simulink model "qvmbocsh41_od_2"  (Simulink 5.0)
settings: Solver=ode45  StartTime=0.0  StopTime=5.0  MaxStep=0.001  RelTol=1e-4
undefined symbols (not defined in the file or in its folder): Z10
libraries: simulink_extras x7, dtlib x1
settings Model: LastModifiedBy=krangelo

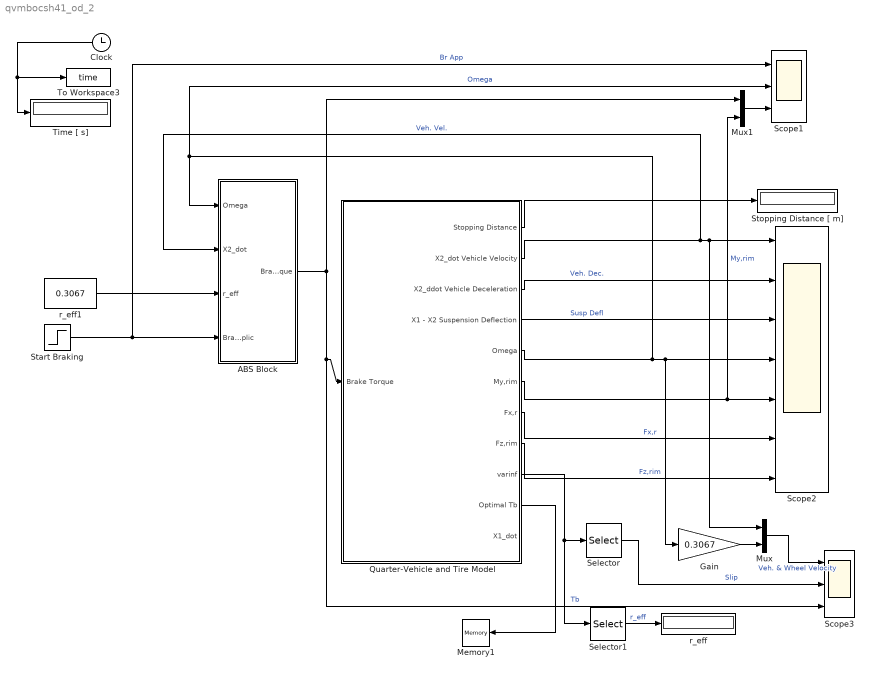
== system qvmbocsh41_od_2 ==
  ABS Block : Subsystem  mask{R1=19000, R2=19000, Bmax=2500, TO=0.0065, TC=0.050, Slip=20, Slipmin=17, neg_a=60, pos_a=3, A=10, om_dot_om=3.5}
      mask prompts: R1 "R1 - Rate of incerase of the  Breake Torque. [Nm/s]"; R2 "R2 - Rate of decerase of the  Breake Torque. [Nm/s]"; Bmax "Bmax - Max. Value of the Brake Torque. [Nm]"; TO "TO - Inlet Valve open time [s]"; TC "TC - Inlet Valve close time [s]"; Slip "Desired slip [%]"; Slipmin "Slipmin - Minimum slip level"; neg_a "-a - Threshold value of the wheel peripheral deceleration [m/s^2]"; pos_a "+a - Threshold value of the wheel peripheral acceleration [m/s^2]"; A "A - Threshold value of the wheel peripheral acceleration [m/s^2]"; om_dot_om "Omdot/Omega -Threshold value of the ratio Om_dot / Om [Hz]"
  Clock : Clock
      settings: Decimation=10
  Gain : Gain  Gain=0.3067  SaturateOnIntegerOverflow=on
  Memory1 : Memory  Orientation=left  X0=0.65
  Mux : Mux  Inputs=2
  Mux1 : Mux  Inputs=2
  Quarter-Vehicle and Tire Model : Subsystem  mask{m2=300, m1=35, kz=20000, Cz=2000, kx=80000, Cx=1100, Vstop=1, Ip=1.04, ro=0.3135, r_eff=0.3067, Vin=80/3.6}
      mask prompts: m2 "m2 - Quarter of the vehicle mass [kg]"; m1 "m1 - Axle mass [kg]"; kz "kz - Suspension stiffness [N/m]"; Cz "cz - Suspension damping [N.s/m]"; kx "kx - Longitudinal suspension stiffness [N/m]"; Cx "cx - Longitudinal suspension damping [N.s/m]"; Vstop "Vstop - Velocity at which the vehicle is considered stoped [m/s]"; Ip "Ip - Wheel polar moment of inertia [kg.m^2]"; ro "ro - Unloaded tire radius [m]"; r_eff "r_eff - Effecive rolling radius [m]"; Vin "Vin - Initial vehicle velocity [m/s]"
      mask help: Vstop - The velocity value, at which the vehicle is considered stoped.
      mask init:
      | disp('initial conditions...')
      | Z10=ro - 9.81*(m1+m2)/195000
      | Z20=Z10 - 9.81*m2/kz
      | X20=0
      | X10=X20+0.01
      | Vin
      | r_eff
      | Om_in=Vin/r_eff
  Scope1 : Scope  NumInputPorts=3
      settings: YMin=0~0~0  YMax=1~95~20000
  Scope2 : Scope  NumInputPorts=7
      settings: TimeRange=5  YMin=21.1325~-1.75e-005~-7e-008~68.8999~0.00025~-0.006~3286.34  YMax=23.3569~0~-6.61744e-024~76.1525~0.00175~0~3286.35  SaveName=ScopeData4
  Scope3 : Scope  NumInputPorts=3
      settings: TimeRange=3  YMin=13.5~-0.225~0  YMax=22.5~0.025~1300  SaveName=ScopeData3
  Selector : Selector  Elements=2  InputPortWidth=40
  Selector1 : Selector  Elements=12  InputPortWidth=40
  Start Braking : Step  Time=2.5  SampleTime=0
  Stopping Distance [ m] : Display
  Time [ s] : Display
  To Workspace3 : ToWorkspace  VariableName=time  SaveFormat=Array
      settings: MaxDataPoints=10000
  r_eff : Display
  r_eff1 : Constant  Value=0.3067
  wires:
  Clock/1 -> Time [ s]/1, To Workspace3/1
  Start Braking/1 -> Scope1/1, ABS Block/4(Brake Applic)  "Br App"
  Quarter-Vehicle and Tire Model/1(Stopping Distance) -> Stopping Distance [ m]/1
  Quarter-Vehicle and Tire Model/5(Omega) -> Scope1/2, ABS Block/1(Omega), Scope2/4, Gain/1  "Omega"
  Quarter-Vehicle and Tire Model/4("X1 - X2 Suspension Deflection ") -> Scope2/3  "Susp Defl"
  Quarter-Vehicle and Tire Model/3(X2_ddot Vehicle Deceleration) -> Scope2/2  "Veh. Dec."
  Quarter-Vehicle and Tire Model/8(Fz,rim) -> Scope2/7  "Fz,rim"
  Quarter-Vehicle and Tire Model/6(My,rim) -> Scope2/5, Mux1/2  "My,rim"
  Quarter-Vehicle and Tire Model/2(X2_dot Vehicle Velocity) -> Scope2/1, Mux/1, ABS Block/2(X2_dot)  "Veh. Vel."
  Quarter-Vehicle and Tire Model/7(Fx,r) -> Scope2/6  "Fx,r"
  ABS Block/1(Brake Torque) -> Scope3/3, Quarter-Vehicle and Tire Model/1(" Brake Torque"), Mux1/1  "Tb"
  Gain/1 -> Mux/2
  Quarter-Vehicle and Tire Model/9(varinf) -> Selector/1, Selector1/1
  Selector/1 -> Scope3/2  "Slip"
  Mux/1 -> Scope3/1  "Veh. & Wheel Velocity"
  Selector1/1 -> r_eff/1  "r_eff"
  r_eff1/1 -> ABS Block/3(r_eff)
  Mux1/1 -> Scope1/3
  Quarter-Vehicle and Tire Model/10(Optimal Tb) -> Memory1/1

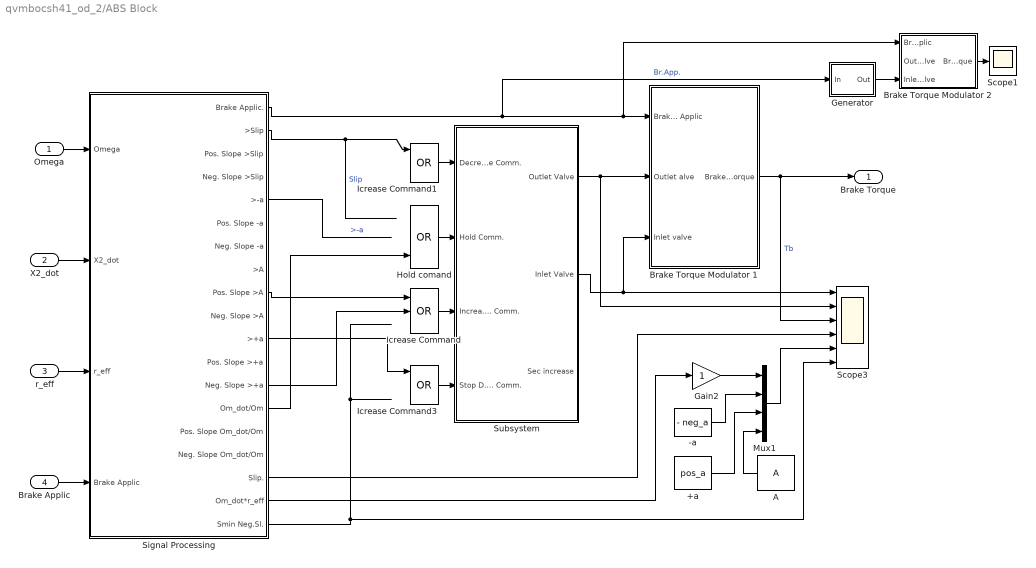
== system qvmbocsh41_od_2/ABS Block ==
  Omega : Inport
  X2_dot : Inport  Port=2
  r_eff : Inport  Port=3
  Brake Applic : Inport  Port=4
  +a : Constant  Value=pos_a
  -a : Constant  Value=- neg_a
  A : Constant  Orientation=left  Value=A
  Brake Torque Modulator 1 : Subsystem  Description=The sysytem holds the Brake Torque at the reached value if no control signal applied  mask{Bmax=Bmax, R1=R1, R2=R2}
      mask prompts: Bmax "Bmax - Max. Value of the Brake Torque. [Nm]"; R1 "R1 - Rate of incerase of the  Brake Torque. [Nm/s]"; R2 "R2 - Rate of decerase of the  Brake Torque. [Nm/s]"
  Brake Torque Modulator 2 : Subsystem  Description=The sysytem holds the Brake Torque at the reached value if no control signal applied  mask{Bmax=Bmax, R1=R1, R2=R2}
      mask prompts: Bmax "Bmax - Max. Value of the Brake Torque. [Nm]"; R1 "R1 - Rate of incerase of the  Brake Torque. [Nm/s]"; R2 "R2 - Rate of decerase of the  Brake Torque. [Nm/s]"
  Gain2 : Gain  SaturateOnIntegerOverflow=on
  Generator : Subsystem  mask{TO=TO, TC=TC}
      mask prompts: TO "Valve open [s]"; TC "Valve closed [s]"
  Hold comand : Logic  Operator=OR  Inputs=3
  Icrease Command : Logic  Operator=OR  Inputs=3
  Icrease Command1 : Logic  Operator=OR  Inputs=3
  Icrease Command3 : Logic  Operator=OR  Inputs=3
  Mux1 : Mux
  Scope1 : Scope
      settings: TimeRange=3  YMin=-1  YMax=1  SaveName=ScopeData5
  Scope3 : Scope  NumInputPorts=6
      settings: TimeRange=3  YMin=0~0~0~-0.025~-90~-5  YMax=1~1~1500~0.225~30~5
  Signal Processing : Subsystem
  Subsystem : Subsystem
  Brake Torque : Outport
  wires:
  Brake Torque Modulator 1/1(Brake Torque) -> Scope3/3, Brake Torque/1  "Tb"
  Subsystem/1(Outlet Valve) -> Scope3/2, Brake Torque Modulator 1/2(Outlet alve)
  Subsystem/2(Inlet Valve) -> Scope3/1, Brake Torque Modulator 1/3(Inlet valve)
  Mux1/1 -> Scope3/5
  A/1 -> Mux1/4
  +a/1 -> Mux1/3
  -a/1 -> Mux1/2
  Gain2/1 -> Mux1/1
  Brake Applic/1 -> Signal Processing/4(Brake Applic)
  Omega/1 -> Signal Processing/1(Omega)
  X2_dot/1 -> Signal Processing/2(X2_dot)
  r_eff/1 -> Signal Processing/3(r_eff)
  Signal Processing/5(>-a) -> ?  ">-a"
  Signal Processing/1(Brake Applic.) -> Generator/1(In), Brake Torque Modulator 1/1(Brake Applic), Brake Torque Modulator 2/1(Brake Applic)  "Br.App."
  Signal Processing/18(" Om_dot*r_eff") -> Gain2/1
  Signal Processing/17(Slip.) -> Scope3/4
  Signal Processing/11(>+a) -> Icrease Command3/1
  Signal Processing/13(Neg. Slope >+a) -> Icrease Command/2
  Signal Processing/14(Om_dot/Om) -> Hold comand/3
  Signal Processing/9(Pos. Slope >A) -> Icrease Command/1
  Signal Processing/2(>Slip) -> Icrease Command1/1  "Slip"
  Hold comand/1 -> Subsystem/2(Hold Comm.)
  Icrease Command/1 -> Subsystem/3(Increase. Comm.)
  Generator/1(Out) -> Brake Torque Modulator 2/3(Inlet valve)
  Brake Torque Modulator 2/1(Brake Torque) -> Scope1/1
  Signal Processing/19(Smin Neg.Sl.) -> Scope3/6
  Icrease Command1/1 -> Subsystem/1(Decrease Comm.)
  Icrease Command3/1 -> Subsystem/4(Stop Dec. Comm.)

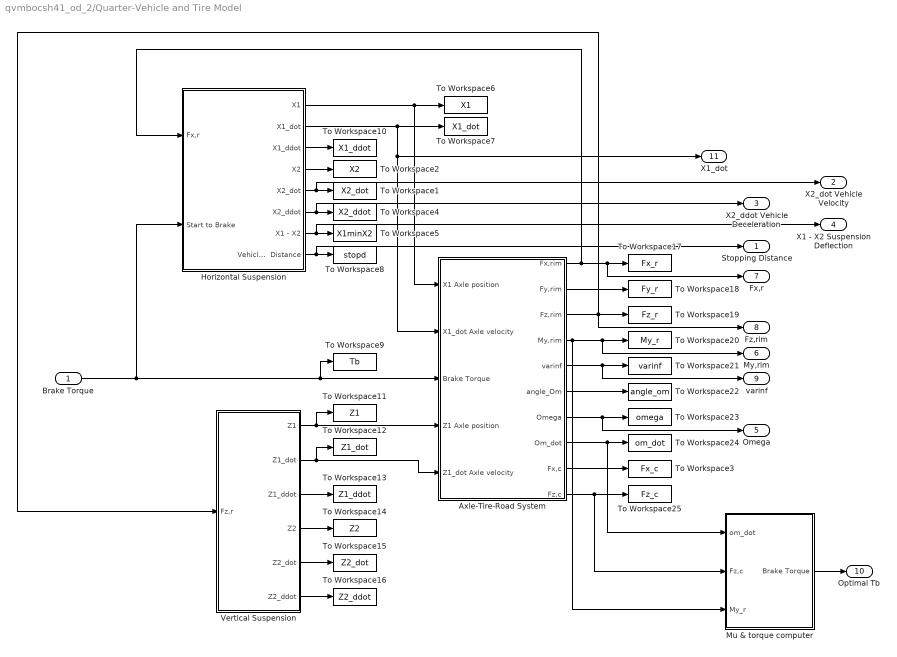
== system qvmbocsh41_od_2/Quarter-Vehicle and Tire Model ==
  " Brake Torque" : Inport
  "Axle-Tire-Road System  " : Subsystem
  Horizontal Suspension : Subsystem
  Mu & torque computer : Subsystem
  To Workspace1 : ToWorkspace  VariableName=X2_dot  SaveFormat=Array
      settings: MaxDataPoints=10000
  To Workspace10 : ToWorkspace  VariableName=X1_ddot  SaveFormat=Array
      settings: MaxDataPoints=10000
  To Workspace11 : ToWorkspace  VariableName=Z1  SaveFormat=Array
      settings: MaxDataPoints=10000
  To Workspace12 : ToWorkspace  VariableName=Z1_dot  SaveFormat=Array
      settings: MaxDataPoints=10000
  To Workspace13 : ToWorkspace  VariableName=Z1_ddot  SaveFormat=Array
      settings: MaxDataPoints=10000
  To Workspace14 : ToWorkspace  VariableName=Z2  SaveFormat=Array
      settings: MaxDataPoints=10000
  To Workspace15 : ToWorkspace  VariableName=Z2_dot  SaveFormat=Array
      settings: MaxDataPoints=10000
  To Workspace16 : ToWorkspace  VariableName=Z2_ddot  SaveFormat=Array
      settings: MaxDataPoints=10000
  To Workspace17 : ToWorkspace  VariableName=Fx_r  SaveFormat=Array
      settings: MaxDataPoints=10000
  To Workspace18 : ToWorkspace  VariableName=Fy_r  SaveFormat=Array
      settings: MaxDataPoints=10000
  To Workspace19 : ToWorkspace  VariableName=Fz_r  SaveFormat=Array
      settings: MaxDataPoints=10000
  To Workspace2 : ToWorkspace  VariableName=X2  SaveFormat=Array
      settings: MaxDataPoints=10000
  To Workspace20 : ToWorkspace  VariableName=My_r  SaveFormat=Array
      settings: MaxDataPoints=10000
  To Workspace21 : ToWorkspace  VariableName=varinf  SaveFormat=Array
      settings: MaxDataPoints=10000
  To Workspace22 : ToWorkspace  VariableName=angle_om  SaveFormat=Array
      settings: MaxDataPoints=10000
  To Workspace23 : ToWorkspace  VariableName=omega  SaveFormat=Array
      settings: MaxDataPoints=10000
  To Workspace24 : ToWorkspace  VariableName=om_dot  SaveFormat=Array
      settings: MaxDataPoints=10000
  To Workspace25 : ToWorkspace  VariableName=Fz_c  SaveFormat=Array
      settings: MaxDataPoints=10000
  To Workspace3 : ToWorkspace  VariableName=Fx_c  SaveFormat=Array
      settings: MaxDataPoints=10000
  To Workspace4 : ToWorkspace  VariableName=X2_ddot  SaveFormat=Array
      settings: MaxDataPoints=10000
  To Workspace5 : ToWorkspace  VariableName=X1minX2  SaveFormat=Array
      settings: MaxDataPoints=10000
  To Workspace6 : ToWorkspace  VariableName=X1  SaveFormat=Array
      settings: MaxDataPoints=10000
  To Workspace7 : ToWorkspace  VariableName=X1_dot  SaveFormat=Array
      settings: MaxDataPoints=10000
  To Workspace8 : ToWorkspace  VariableName=stopd  SaveFormat=Array
      settings: MaxDataPoints=10000
  To Workspace9 : ToWorkspace  VariableName=Tb  SaveFormat=Array
      settings: MaxDataPoints=10000
  Vertical Suspension : Subsystem
  Stopping Distance : Outport
  X2_dot Vehicle Velocity : Outport  Port=2
  X2_ddot Vehicle Deceleration : Outport  Port=3
  "X1 - X2 Suspension Deflection " : Outport  Port=4
  Omega : Outport  Port=5
  My,rim : Outport  Port=6
  Fx,r : Outport  Port=7
  Fz,rim : Outport  Port=8
  varinf : Outport  Port=9
  Optimal Tb : Outport  Port=10
  X1_dot : Outport  Port=11
  wires:
  "Axle-Tire-Road System  "/1(Fx,rim) -> Horizontal Suspension/1("Fx,r "), To Workspace17/1, Fx,r/1
  "Axle-Tire-Road System  "/3(Fz,rim) -> To Workspace19/1, Vertical Suspension/1("Fz,r "), Fz,rim/1
  Horizontal Suspension/1(X1) -> "Axle-Tire-Road System  "/1(X1 Axle position), To Workspace6/1
  Vertical Suspension/1(Z1) -> To Workspace11/1, "Axle-Tire-Road System  "/4(Z1 Axle position)
  Vertical Suspension/2(Z1_dot) -> To Workspace12/1, "Axle-Tire-Road System  "/5(Z1_dot Axle velocity)
  Horizontal Suspension/2(X1_dot) -> To Workspace7/1, "Axle-Tire-Road System  "/2(X1_dot Axle velocity), X1_dot/1
  " Brake Torque"/1 -> "Axle-Tire-Road System  "/3(Brake Torque), To Workspace9/1, Horizontal Suspension/2(Start to Brake)
  Horizontal Suspension/8("Vehicle Stopping  Distance ") -> To Workspace8/1, Stopping Distance/1
  Horizontal Suspension/3(X1_ddot) -> To Workspace10/1
  Horizontal Suspension/4(X2) -> To Workspace2/1
  Horizontal Suspension/5(X2_dot) -> To Workspace1/1, X2_dot Vehicle Velocity/1
  Horizontal Suspension/6(X2_ddot) -> To Workspace4/1, X2_ddot Vehicle Deceleration/1
  Horizontal Suspension/7(X1 - X2) -> To Workspace5/1, "X1 - X2 Suspension Deflection "/1
  Vertical Suspension/3(Z1_ddot) -> To Workspace13/1
  Vertical Suspension/4(Z2) -> To Workspace14/1
  Vertical Suspension/5(Z2_dot) -> To Workspace15/1
  Vertical Suspension/6(Z2_ddot) -> To Workspace16/1
  "Axle-Tire-Road System  "/2(Fy,rim) -> To Workspace18/1
  "Axle-Tire-Road System  "/4(My,rim) -> To Workspace20/1, My,rim/1, Mu & torque computer/3(My_r)
  "Axle-Tire-Road System  "/5(varinf) -> To Workspace21/1, varinf/1
  "Axle-Tire-Road System  "/6(angle_Om) -> To Workspace22/1
  "Axle-Tire-Road System  "/7(" Omega") -> To Workspace23/1, Omega/1
  "Axle-Tire-Road System  "/8(Om_dot) -> To Workspace24/1, Mu & torque computer/1(om_dot)
  "Axle-Tire-Road System  "/9(Fx,c) -> To Workspace3/1
  "Axle-Tire-Road System  "/10(Fz,c) -> To Workspace25/1, Mu & torque computer/2(Fz,c)
  Mu & torque computer/1(Brake Torque) -> Optimal Tb/1

== system qvmbocsh41_od_2/ABS Block/Brake Torque Modulator 1 ==
  Brake Applic : Inport
  Outlet alve : Inport  Port=2
  Inlet valve : Inport  Port=3
  Constant2 : Constant  Orientation=left  Value=0
  Integrator : Integrator  LimitOutput=on  UpperSaturationLimit=Bmax  LowerSaturationLimit=0
  Rate of Increase : Constant  Orientation=left  Value=R1
  Rate of decrease : Constant  Orientation=left  Value=R2
  Sum : Sum  Inputs=|+-  SaturateOnIntegerOverflow=on  InputSameDT=on
  Switch : Switch  Threshold=1  SaturateOnIntegerOverflow=on  InputSameDT=on
  Switch1 : Switch  Threshold=1  SaturateOnIntegerOverflow=on  InputSameDT=on
  Switch2 : Switch  Threshold=1  SaturateOnIntegerOverflow=on  InputSameDT=on
  Brake Torque : Outport
  wires:
  Switch/1 -> Switch2/1
  Brake Applic/1 -> Switch2/2
  Switch2/1 -> Sum/1
  Rate of decrease/1 -> Switch1/1
  Rate of Increase/1 -> Switch/3
  Switch1/1 -> Sum/2
  Integrator/1 -> Brake Torque/1
  Outlet alve/1 -> Switch1/2
  Inlet valve/1 -> Switch/2
  Constant2/1 -> Switch2/3, Switch1/3, Switch/1
  Sum/1 -> Integrator/1

== system qvmbocsh41_od_2/ABS Block/Brake Torque Modulator 2 ==
  Brake Applic : Inport
  Outlet alve : Inport  Port=2
  Inlet valve : Inport  Port=3
  Constant2 : Constant  Orientation=left  Value=0
  Integrator : Integrator  LimitOutput=on  UpperSaturationLimit=Bmax  LowerSaturationLimit=0
  Rate of Increase : Constant  Orientation=left  Value=R1
  Rate of decrease : Constant  Orientation=left  Value=R2
  Sum : Sum  Inputs=|+-  SaturateOnIntegerOverflow=on  InputSameDT=on
  Switch : Switch  Threshold=1  SaturateOnIntegerOverflow=on  InputSameDT=on
  Switch1 : Switch  Threshold=1  SaturateOnIntegerOverflow=on  InputSameDT=on
  Switch2 : Switch  Threshold=1  SaturateOnIntegerOverflow=on  InputSameDT=on
  Brake Torque : Outport
  wires:
  Switch/1 -> Switch2/1
  Brake Applic/1 -> Switch2/2
  Switch2/1 -> Sum/1
  Rate of decrease/1 -> Switch1/1
  Rate of Increase/1 -> Switch/3
  Switch1/1 -> Sum/2
  Integrator/1 -> Brake Torque/1
  Outlet alve/1 -> Switch1/2
  Inlet valve/1 -> Switch/2
  Constant2/1 -> Switch2/3, Switch1/3, Switch/1
  Sum/1 -> Integrator/1

== system qvmbocsh41_od_2/ABS Block/Generator ==
  In : Inport
  Constant1 : Constant  Orientation=left  Value=0
  Data Type Conversion1 : DataTypeConversion  DataType=boolean  SaturateOnIntegerOverflow=on
  Data Type Conversion2 : DataTypeConversion  Orientation=left  DataType=double  SaturateOnIntegerOverflow=on
  Data Type Conversion5 : DataTypeConversion  DataType=boolean  SaturateOnIntegerOverflow=on
  Logical Operator2 : Logic  Operator=OR
  Memory1 : Memory  Orientation=left
  Memory2 : Memory  Orientation=left
  Subsystem2 : Subsystem
  Switch2 : Switch  Threshold=1  SaturateOnIntegerOverflow=on  InputSameDT=on
  Timer R1 : Subsystem  mask{TC=TC}
      mask prompts: TC "Cycle Time [s]"
  Timer R2 : Subsystem  mask{TO=TO}
      mask prompts: TO "Open time [s]"
  Out : Outport
  wires:
  Timer R2/1(Time elapse) -> Out/1
  Data Type Conversion2/1 -> Switch2/1
  Data Type Conversion1/1 -> Logical Operator2/2
  Constant1/1 -> Switch2/3
  Memory2/1 -> Data Type Conversion2/1
  Switch2/1 -> Data Type Conversion1/1
  Memory1/1 -> Memory2/1, Timer R2/2(Reset), Timer R1/2(Reset)
  Data Type Conversion5/1 -> Switch2/2, Subsystem2/1(In1)
  Subsystem2/1(Pos. Slpoe) -> Logical Operator2/1
  In/1 -> Data Type Conversion5/1
  Timer R1/1(Time elapse) -> Memory1/1
  Logical Operator2/1 -> Timer R1/1(Start), Timer R2/1(Start)

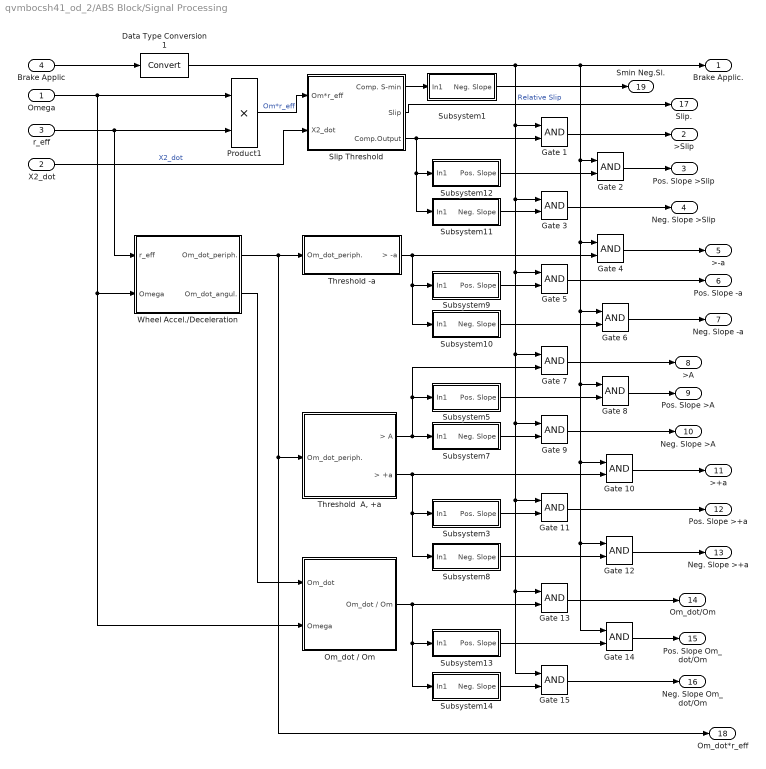
== system qvmbocsh41_od_2/ABS Block/Signal Processing ==
  Omega : Inport
  X2_dot : Inport  Port=2
  r_eff : Inport  Port=3
  Brake Applic : Inport  Port=4
  " Wheel Accel./Deceleration" : Subsystem
  Data Type Conversion1 : DataTypeConversion  DataType=boolean  SaturateOnIntegerOverflow=on
  Gate {1..15} (15 alike) : Logic
  Om_dot / Om : Subsystem
  Product1 : Product  Inputs=**  SaturateOnIntegerOverflow=on  InputSameDT=on
  Slip Threshold : Subsystem
  Subsystem1 : Subsystem
  Subsystem10 : Subsystem
  Subsystem11 : Subsystem
  Subsystem12 : Subsystem
  Subsystem13 : Subsystem
  Subsystem14 : Subsystem
  Subsystem3 : Subsystem
  Subsystem5 : Subsystem
  Subsystem7 : Subsystem
  Subsystem8 : Subsystem
  Subsystem9 : Subsystem
  "Threshold  A, +a" : Subsystem
  Threshold -a : Subsystem
  Brake Applic. : Outport
  >Slip : Outport  Port=2
  Pos. Slope >Slip : Outport  Port=3
  Neg. Slope >Slip : Outport  Port=4
  >-a : Outport  Port=5
  Pos. Slope -a : Outport  Port=6
  Neg. Slope -a : Outport  Port=7
  >A : Outport  Port=8
  Pos. Slope >A : Outport  Port=9
  "Neg. Slope >A " : Outport  Port=10
  >+a : Outport  Port=11
  Pos. Slope >+a : Outport  Port=12
  Neg. Slope >+a : Outport  Port=13
  Om_dot/Om : Outport  Port=14
  Pos. Slope Om_dot/Om : Outport  Port=15
  Neg. Slope Om_dot/Om : Outport  Port=16
  Slip. : Outport  Port=17
  " Om_dot*r_eff" : Outport  Port=18
  Smin Neg.Sl. : Outport  Port=19
  wires:
  Brake Applic/1 -> Data Type Conversion1/1
  Product1/1 -> Slip Threshold/1(Om*r_eff)  "Om*r_eff"
  X2_dot/1 -> Slip Threshold/2(X2_dot)  "X2_dot"
  r_eff/1 -> Product1/2, " Wheel Accel./Deceleration"/1(r_eff)
  Omega/1 -> Om_dot / Om/2(Omega), " Wheel Accel./Deceleration"/2(Omega), Product1/1
  "Threshold  A, +a"/1(" > A") -> Subsystem7/1(In1), Subsystem5/1(In1), Gate 7/2
  "Threshold  A, +a"/2(> +a) -> Subsystem3/1(In1), Subsystem8/1(In1), Gate 10/2
  Subsystem8/1(Neg. Slope) -> Gate 12/2
  Subsystem3/1(Pos. Slope) -> Gate 11/2
  Subsystem7/1(Neg. Slope) -> Gate 9/2
  Subsystem5/1(Pos. Slope) -> Gate 8/2
  Subsystem10/1(Neg. Slope) -> Gate 6/2
  Subsystem9/1(Pos. Slope) -> Gate 5/2
  Threshold -a/1(> -a) -> Subsystem10/1(In1), Subsystem9/1(In1), Gate 4/2
  Subsystem11/1(Neg. Slope) -> Gate 3/2
  Subsystem12/1(Pos. Slope) -> Gate 2/2
  Slip Threshold/3(Comp.Output) -> Subsystem12/1(In1), Subsystem11/1(In1), Gate 1/2
  Om_dot / Om/1(Om_dot / Om) -> Subsystem13/1(In1), Subsystem14/1(In1), Gate 13/2
  Subsystem14/1(Neg. Slope) -> Gate 15/2
  Subsystem13/1(Pos. Slope) -> Gate 14/2
  Data Type Conversion1/1 -> Gate 1/1, Gate 3/1, Gate 5/1, Gate 7/1, Gate 9/1, Gate 11/1, Gate 13/1, Gate 15/1, Brake Applic./1, Gate 2/1, Gate 4/1, Gate 6/1, Gate 8/1, Gate 10/1, Gate 12/1, Gate 14/1
  Gate 1/1 -> >Slip/1
  Gate 2/1 -> Pos. Slope >Slip/1
  Gate 3/1 -> Neg. Slope >Slip/1
  Gate 4/1 -> >-a/1
  Gate 5/1 -> Pos. Slope -a/1
  Gate 6/1 -> Neg. Slope -a/1
  Gate 7/1 -> >A/1
  Gate 8/1 -> Pos. Slope >A/1
  Gate 9/1 -> "Neg. Slope >A "/1
  Gate 10/1 -> >+a/1
  Gate 11/1 -> Pos. Slope >+a/1
  Gate 13/1 -> Om_dot/Om/1
  Gate 14/1 -> Pos. Slope Om_dot/Om/1
  Gate 15/1 -> Neg. Slope Om_dot/Om/1
  " Wheel Accel./Deceleration"/1(Om_dot_periph.) -> " Om_dot*r_eff"/1, "Threshold  A, +a"/1(Om_dot_periph.), Threshold -a/1(Om_dot_periph.)
  Gate 12/1 -> Neg. Slope >+a/1
  Slip Threshold/2(Slip) -> Slip./1  "Relative Slip"
  " Wheel Accel./Deceleration"/2(Om_dot_angul.) -> Om_dot / Om/1(Om_dot)
  Slip Threshold/1(Comp. S-min) -> Subsystem1/1(In1)
  Subsystem1/1(Neg. Slope) -> Smin Neg.Sl./1

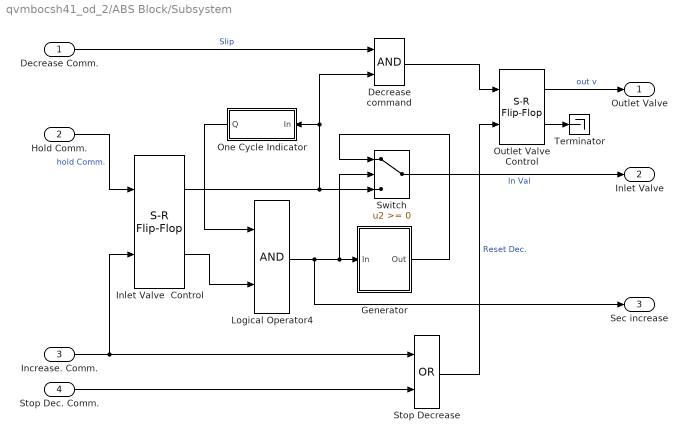
== system qvmbocsh41_od_2/ABS Block/Subsystem ==
  Decrease Comm. : Inport
  Hold Comm. : Inport  Port=2
  Increase. Comm. : Inport  Port=3
  Stop Dec. Comm. : Inport  Port=4
  Decrease command : Logic
  Generator : Subsystem  mask{TO=TO, TC=TC}
      mask prompts: TO "Valve open [s]"; TC "Valve closed [s]"
  Inlet Valve  Control : simulink_extras/Flip Flops/S-R Flip-Flop  initial_condition=0
  Logical Operator4 : Logic
  One Cycle Indicator : Subsystem  Orientation=left
  Outlet Valve Control : simulink_extras/Flip Flops/S-R Flip-Flop  initial_condition=0
  Stop Decrease : Logic  Operator=OR
  Switch : Switch  SaturateOnIntegerOverflow=on  InputSameDT=on
  Terminator : Terminator
  Outlet Valve : Outport
  Inlet Valve : Outport  Port=2
  Sec increase : Outport  Port=3
  wires:
  Decrease command/1 -> Outlet Valve Control/1
  Inlet Valve  Control/1 -> Switch/3, Decrease command/2, One Cycle Indicator/1(In)
  Stop Decrease/1 -> Outlet Valve Control/2  "Reset Dec."
  Logical Operator4/1 -> Generator/1(In), Switch/2, Sec increase/1
  Inlet Valve  Control/2 -> Logical Operator4/2
  Generator/1(Out) -> Switch/1
  Decrease Comm./1 -> Decrease command/1  "Slip"
  Outlet Valve Control/1 -> Outlet Valve/1  "out v"
  Hold Comm./1 -> Inlet Valve  Control/1  "hold Comm."
  Switch/1 -> Inlet Valve/1  "In Val"
  Increase. Comm./1 -> Inlet Valve  Control/2, Stop Decrease/1
  Stop Dec. Comm./1 -> Stop Decrease/2
  One Cycle Indicator/1(Q) -> Logical Operator4/1
  Outlet Valve Control/2 -> Terminator/1

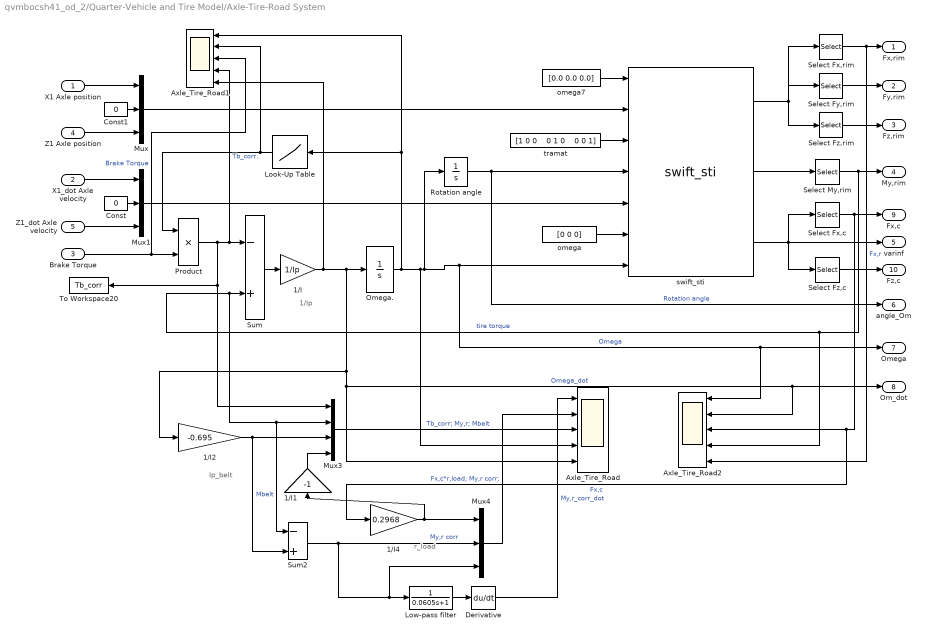
== system qvmbocsh41_od_2/Quarter-Vehicle and Tire Model/Axle-Tire-Road System   ==
  note: 1/Ip
  note: r_load
  note: Ip_belt
  X1 Axle position : Inport
  X1_dot Axle velocity : Inport  Port=2
  Brake Torque : Inport  Port=3
  Z1 Axle position : Inport  Port=4
  Z1_dot Axle velocity : Inport  Port=5
  1/I : Gain  Gain=1/Ip  SaturateOnIntegerOverflow=on
  1/I1 : Gain  Orientation=up  Gain=-1  SaturateOnIntegerOverflow=on
  1/I2 : Gain  Gain=-0.695  SaturateOnIntegerOverflow=on
  1/I4 : Gain  Gain=0.2968  SaturateOnIntegerOverflow=on
  Axle_Tire_Road : Scope  NumInputPorts=5
      settings: YMin=-25000~-1500~-250~35~-250  YMax=10000~250~1500~75~200  SaveName=ScopeData8
  Axle_Tire_Road1 : Scope  NumInputPorts=5
      settings: YMin=0~5.55112e-017~0~0~-1500  YMax=100~1.1~9000~3500~250  SaveName=ScopeData9
  Axle_Tire_Road2 : Scope  NumInputPorts=5
      settings: YMin=0~-1500~-5000~-250~-5000  YMax=80~250~1000~1750~1000  SaveName=ScopeData2
  Const : Constant  Value=0
  Const1 : Constant  Value=0
  Derivative : Derivative
  Look-Up Table : Lookup  Orientation=left  InputValues=[-10:0.01:10]  OutputValues=tanh(0.5*[-10:0.01:10])  SaturateOnIntegerOverflow=on
  Low-pass filter : TransferFcn  Denominator=[0.0605 1]
  Mux : Mux  Inputs=3
  Mux1 : Mux  Inputs=3
  Mux3 : Mux
  Mux4 : Mux  Inputs=3
  Omega. : Integrator  InitialCondition=Om_in  UpperSaturationLimit=200  LowerSaturationLimit=0
  Product : Product  SaturateOnIntegerOverflow=on  InputSameDT=on
  Rotation angle : Integrator  UpperSaturationLimit=1000  LowerSaturationLimit=0
  Select Fx,c : Selector  Elements=4  InputPortWidth=40
  Select Fx,rim : Selector  InputPortWidth=3
  Select Fy,rim : Selector  Elements=2  InputPortWidth=3
  Select Fz,c : Selector  Elements=6  InputPortWidth=40
  Select Fz,rim : Selector  Elements=3  InputPortWidth=3
  Select My,rim : Selector  Elements=2  InputPortWidth=3
  Sum : Sum  Inputs=-+  SaturateOnIntegerOverflow=on  InputSameDT=on
  Sum2 : Sum  Inputs=-+  SaturateOnIntegerOverflow=on  InputSameDT=on
  To Workspace20 : ToWorkspace  VariableName=Tb_corr  SaveFormat=Array
      settings: MaxDataPoints=10000
  omega : Constant  Value=[0 0 0]
  omega7 : Constant  Value=[0.0 0.0 0.0]
  swift_sti : dtlib/swift_sti  idtyre=1  use_mode=124  tpfname='L_swt_car205_60R15.tir'  road_popup=Data file (effective inputs)  rdfname='div_road_5.rdf'
  tramat : Constant  Value="[1 0 0    0 1 0    0 0 1]"
  Fx,rim : Outport
  Fy,rim : Outport  Port=2
  Fz,rim : Outport  Port=3
  My,rim : Outport  Port=4
  varinf : Outport  Port=5
  angle_Om : Outport  Port=6
  " Omega" : Outport  Port=7
  Om_dot : Outport  Port=8
  Fx,c : Outport  Port=9
  Fz,c : Outport  Port=10
  wires:
  1/I/1 -> Omega./1, Axle_Tire_Road2/2, Om_dot/1, Axle_Tire_Road/5, 1/I2/1, Axle_Tire_Road1/5  "Omega_dot"
  Omega./1 -> Rotation angle/1, swift_sti/7, " Omega"/1, Axle_Tire_Road2/1, Axle_Tire_Road/4, Axle_Tire_Road1/1, Look-Up Table/1  "Omega"
  omega7/1 -> swift_sti/1
  tramat/1 -> swift_sti/3
  omega/1 -> swift_sti/6
  Rotation angle/1 -> angle_Om/1, swift_sti/4  "Rotation angle"
  Product/1 -> Axle_Tire_Road1/4, Sum/1, Mux3/1, To Workspace20/1  "Tb_corr."
  Look-Up Table/1 -> Axle_Tire_Road1/2, Product/1
  Brake Torque/1 -> Axle_Tire_Road1/3, Product/2  "Brake Torque"
  X1 Axle position/1 -> Mux/1
  Z1 Axle position/1 -> Mux/3
  X1_dot Axle velocity/1 -> Mux1/1
  Z1_dot Axle velocity/1 -> Mux1/3
  swift_sti/1 -> Select Fz,rim/1, Select Fx,rim/1, Select Fy,rim/1
  Select Fy,rim/1 -> Fy,rim/1
  Select Fx,rim/1 -> Fx,rim/1, Axle_Tire_Road2/5  "Fx,r"
  Select Fz,rim/1 -> Fz,rim/1
  swift_sti/3 -> Select Fz,c/1, Select Fx,c/1, varinf/1
  swift_sti/2 -> Select My,rim/1
  Select My,rim/1 -> My,rim/1, Sum/2, Mux3/2, Sum2/1, Axle_Tire_Road2/4  "tire torque"
  Mux1/1 -> swift_sti/5
  Mux/1 -> swift_sti/2
  Sum/1 -> 1/I/1
  Select Fx,c/1 -> Fx,c/1, Axle_Tire_Road2/3, 1/I4/1  "Fx,c"
  Select Fz,c/1 -> Fz,c/1
  Const/1 -> Mux1/2
  Const1/1 -> Mux/2
  Derivative/1 -> Axle_Tire_Road/1  "My,r_corr_dot"
  1/I2/1 -> Mux3/3, Sum2/2  "Mbelt"
  Mux3/1 -> Axle_Tire_Road/3  "Tb_corr; My,r; Mbelt"
  Sum2/1 -> Mux4/2, Mux4/3, Low-pass filter/1  "My,r corr"
  Mux4/1 -> Axle_Tire_Road/2  "Fx,c*r,load; My,r corr;"
  1/I4/1 -> Mux4/1, 1/I1/1
  1/I1/1 -> Mux3/4
  Low-pass filter/1 -> Derivative/1

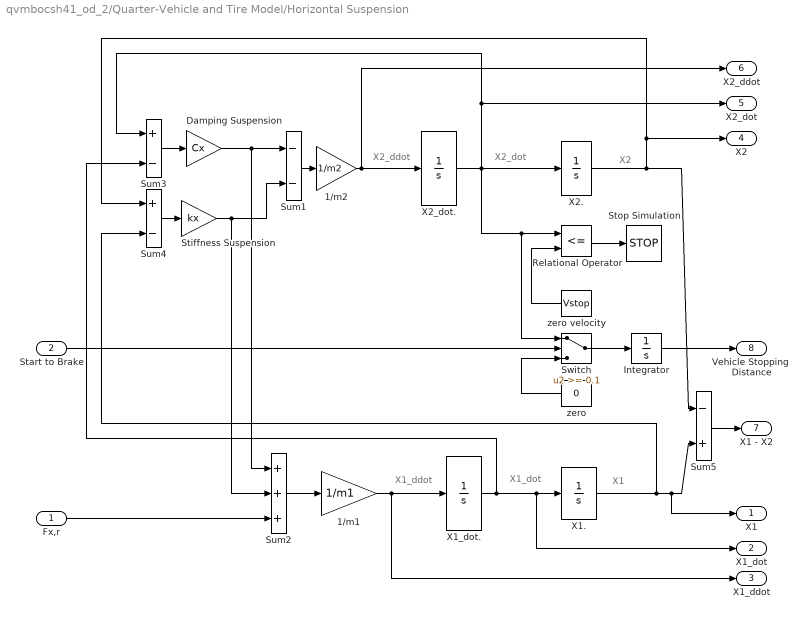
== system qvmbocsh41_od_2/Quarter-Vehicle and Tire Model/Horizontal Suspension ==
  note: X1_dot
  note: X2_dot
  note: X1
  note: X2_ddot
  note: X2
  note: X1_ddot
  "Fx,r " : Inport
  Start to Brake : Inport  Port=2
  1/m1 : Gain  Gain=1/m1  SaturateOnIntegerOverflow=on
  1/m2 : Gain  Gain=1/m2  SaturateOnIntegerOverflow=on
  Damping Suspension : Gain  Gain=Cx  SaturateOnIntegerOverflow=on
  Integrator : Integrator
  Relational Operator : RelationalOperator  Operator=<=  InputSameDT=on
  Stiffness Suspension : Gain  Gain=kx  SaturateOnIntegerOverflow=on
  Stop Simulation : Stop
  Sum1 : Sum  Inputs=--  SaturateOnIntegerOverflow=on  InputSameDT=on
  Sum2 : Sum  Inputs=+++  SaturateOnIntegerOverflow=on  InputSameDT=on
  Sum3 : Sum  Inputs=+-  SaturateOnIntegerOverflow=on  InputSameDT=on
  Sum4 : Sum  Inputs=+-  SaturateOnIntegerOverflow=on  InputSameDT=on
  Sum5 : Sum  Inputs=-+  SaturateOnIntegerOverflow=on  InputSameDT=on
  Switch : Switch  Threshold=0.1  SaturateOnIntegerOverflow=on  InputSameDT=on
  X1. : Integrator  InitialCondition=X10  UpperSaturationLimit=+inf  LowerSaturationLimit=-0.1
  X1_dot. : Integrator  InitialCondition=Vin  UpperSaturationLimit=34  LowerSaturationLimit=0
  X2. : Integrator  InitialCondition=X20
  X2_dot. : Integrator  InitialCondition=Vin  UpperSaturationLimit=34  LowerSaturationLimit=0
  "zero " : Constant  Orientation=left  Value=0
  zero velocity : Constant  Orientation=left  Value=Vstop
  X1 : Outport
  X1_dot : Outport  Port=2
  X1_ddot : Outport  Port=3
  X2 : Outport  Port=4
  X2_dot : Outport  Port=5
  X2_ddot : Outport  Port=6
  X1 - X2 : Outport  Port=7
  "Vehicle Stopping  Distance " : Outport  Port=8
  wires:
  Relational Operator/1 -> Stop Simulation/1
  zero velocity/1 -> Relational Operator/2
  Switch/1 -> Integrator/1
  Stiffness Suspension/1 -> Sum1/2, Sum2/2
  Sum4/1 -> Stiffness Suspension/1
  Sum3/1 -> Damping Suspension/1
  X2./1 -> Sum5/1, Sum4/1, X2/1
  Sum1/1 -> 1/m2/1
  X1_dot./1 -> Sum3/2, X1./1, X1_dot/1
  X1./1 -> Sum4/2, Sum5/2, X1/1
  Sum2/1 -> 1/m1/1
  1/m1/1 -> X1_dot./1, X1_ddot/1
  Damping Suspension/1 -> Sum1/1, Sum2/1
  X2_dot./1 -> Relational Operator/1, Switch/1, X2./1, Sum3/1, X2_dot/1
  1/m2/1 -> X2_dot./1, X2_ddot/1
  "Fx,r "/1 -> Sum2/3
  Sum5/1 -> X1 - X2/1
  Integrator/1 -> "Vehicle Stopping  Distance "/1
  Start to Brake/1 -> Switch/2
  "zero "/1 -> Switch/3

== system qvmbocsh41_od_2/Quarter-Vehicle and Tire Model/Mu & torque computer ==
  note: I_belt
  om_dot : Inport
  Fz,c : Inport  Port=2
  My_r : Inport  Port=3
  1/I2 : Gain  Gain=-0.695  SaturateOnIntegerOverflow=on
  A : Constant  Orientation=left
  Memory1 : Memory  X0=0.65
  Product1 : Product  SaturateOnIntegerOverflow=on  InputSameDT=on
  Product2 : Product  Inputs=*/  SaturateOnIntegerOverflow=on  InputSameDT=on
  Product4 : Product  SaturateOnIntegerOverflow=on  InputSameDT=on
  Scope1 : Scope  NumInputPorts=6
      settings: YMin=950~0.95~1000~950~-100~1000  YMax=1300~1.3~1350~1300~100~1350  SaveName=ScopeData6
  Sum : Sum  SaturateOnIntegerOverflow=on
  Sum1 : Sum  Inputs=+-  SaturateOnIntegerOverflow=on
  r_load : Fcn  Expr=0.3135 - (u(1)/200000)
  Brake Torque : Outport
  wires:
  om_dot/1 -> 1/I2/1
  Fz,c/1 -> Product1/2, r_load/1
  r_load/1 -> Product1/1
  Memory1/1 -> Product4/2
  Product1/1 -> Product4/1, Product2/2
  1/I2/1 -> Sum1/2, Scope1/5, Sum/1
  Sum/1 -> Brake Torque/1, Scope1/3
  My_r/1 -> Sum1/1, Scope1/6
  Sum1/1 -> Product2/1, Scope1/1  "My,r corr"
  Product4/1 -> Sum/2, Scope1/4
  Product2/1 -> Memory1/1, Scope1/2

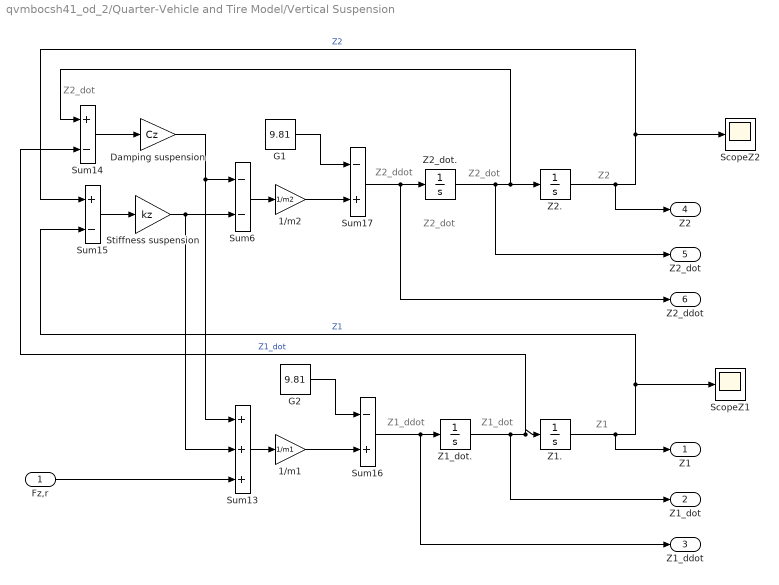
== system qvmbocsh41_od_2/Quarter-Vehicle and Tire Model/Vertical Suspension ==
  note: Z2
  note: Z2_dot
  note: Z1_dot
  note: Z1_ddot
  note: Z2_ddot
  note: Z2_dot
  note: Z2_dot
  note: Z1
  "Fz,r " : Inport
  1/m1 : Gain  Gain=1/m1  SaturateOnIntegerOverflow=on
  1/m2 : Gain  Gain=1/m2  SaturateOnIntegerOverflow=on
  Damping suspension : Gain  Gain=Cz  SaturateOnIntegerOverflow=on
  G1 : Constant  Value=9.81
  G2 : Constant  Value=9.81
  ScopeZ1 : Scope
      settings: YMin=0.3  YMax=0.3225  SaveName=ScopeData11
  ScopeZ2 : Scope
      settings: YMin=0.1  YMax=0.15  SaveName=ScopeData12
  Stiffness suspension : Gain  Gain=kz  SaturateOnIntegerOverflow=on
  Sum13 : Sum  Inputs=+++  SaturateOnIntegerOverflow=on  InputSameDT=on
  Sum14 : Sum  Inputs=+-  SaturateOnIntegerOverflow=on  InputSameDT=on
  Sum15 : Sum  Inputs=+-  SaturateOnIntegerOverflow=on  InputSameDT=on
  Sum16 : Sum  Inputs=-+  SaturateOnIntegerOverflow=on  InputSameDT=on
  Sum17 : Sum  Inputs=-+  SaturateOnIntegerOverflow=on  InputSameDT=on
  Sum6 : Sum  Inputs=--  SaturateOnIntegerOverflow=on  InputSameDT=on
  Z1. : Integrator  InitialCondition=Z10  UpperSaturationLimit=+inf  LowerSaturationLimit=-0.1
  Z1_dot. : Integrator
  Z2. : Integrator  InitialCondition=Z20
  Z2_dot. : Integrator
  Z1 : Outport
  Z1_dot : Outport  Port=2
  Z1_ddot : Outport  Port=3
  Z2 : Outport  Port=4
  Z2_dot : Outport  Port=5
  Z2_ddot : Outport  Port=6
  wires:
  Stiffness suspension/1 -> Sum6/2, Sum13/2
  Sum15/1 -> Stiffness suspension/1
  Sum14/1 -> Damping suspension/1
  Sum6/1 -> 1/m2/1
  Sum17/1 -> Z2_dot./1, Z2_ddot/1
  1/m2/1 -> Sum17/2
  G1/1 -> Sum17/1
  Z1./1 -> Z1/1, Sum15/2, ScopeZ1/1  "Z1"
  Sum16/1 -> Z1_dot./1, Z1_ddot/1
  1/m1/1 -> Sum16/2
  G2/1 -> Sum16/1
  Damping suspension/1 -> Sum6/1, Sum13/1
  Sum13/1 -> 1/m1/1
  Z1_dot./1 -> Z1./1, Sum14/2, Z1_dot/1  "Z1_dot"
  Z2_dot./1 -> Z2./1, Sum14/1, Z2_dot/1
  Z2./1 -> Z2/1, Sum15/1, ScopeZ2/1  "Z2"
  "Fz,r "/1 -> Sum13/3

== system qvmbocsh41_od_2/ABS Block/Generator/Subsystem2 ==
  In1 : Inport
  Logical Operator2 : Logic  Operator=XOR
  Logical Operator3 : Logic
  Memory : Memory
  Pos. Slpoe : Outport
  wires:
  Logical Operator3/1 -> Pos. Slpoe/1
  In1/1 -> Logical Operator3/1, Memory/1, Logical Operator2/2
  Logical Operator2/1 -> Logical Operator3/2
  Memory/1 -> Logical Operator2/1

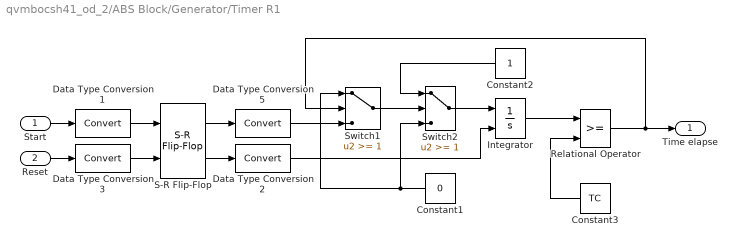
== system qvmbocsh41_od_2/ABS Block/Generator/Timer R1 ==
  Start : Inport
  Reset : Inport  Port=2
  Constant1 : Constant  Orientation=left  Value=0
  Constant2 : Constant  Orientation=left
  Constant3 : Constant  Orientation=left  Value=TC
  Data Type Conversion1 : DataTypeConversion  DataType=boolean  SaturateOnIntegerOverflow=on
  Data Type Conversion2 : DataTypeConversion  DataType=double  SaturateOnIntegerOverflow=on
  Data Type Conversion3 : DataTypeConversion  DataType=boolean  SaturateOnIntegerOverflow=on
  Data Type Conversion5 : DataTypeConversion  DataType=double  SaturateOnIntegerOverflow=on
  Integrator : Integrator  ExternalReset=level
  Relational Operator : RelationalOperator  InputSameDT=on
  S-R Flip-Flop : simulink_extras/Flip Flops/S-R Flip-Flop  initial_condition=0
  Switch1 : Switch  Threshold=1  SaturateOnIntegerOverflow=on  InputSameDT=on
  Switch2 : Switch  Threshold=1  SaturateOnIntegerOverflow=on  InputSameDT=on
  Time elapse : Outport
  wires:
  Data Type Conversion5/1 -> Switch1/3
  S-R Flip-Flop/1 -> Data Type Conversion5/1
  Data Type Conversion2/1 -> Integrator/2
  S-R Flip-Flop/2 -> Data Type Conversion2/1
  Start/1 -> Data Type Conversion1/1
  Data Type Conversion1/1 -> S-R Flip-Flop/1
  Reset/1 -> Data Type Conversion3/1
  Data Type Conversion3/1 -> S-R Flip-Flop/2
  Switch2/1 -> Integrator/1
  Constant3/1 -> Relational Operator/2
  Constant1/1 -> Switch1/1, Switch2/3
  Integrator/1 -> Relational Operator/1
  Relational Operator/1 -> Switch1/2, Time elapse/1
  Switch1/1 -> Switch2/2
  Constant2/1 -> Switch2/1

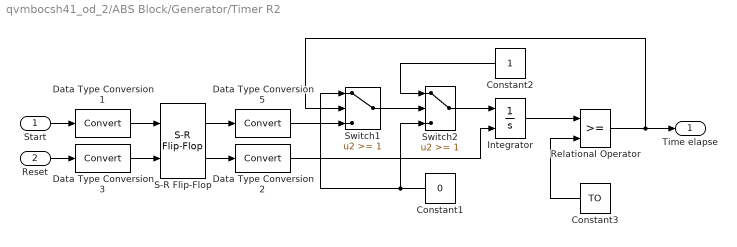
== system qvmbocsh41_od_2/ABS Block/Generator/Timer R2 ==
  Start : Inport
  Reset : Inport  Port=2
  Constant1 : Constant  Orientation=left  Value=0
  Constant2 : Constant  Orientation=left
  Constant3 : Constant  Orientation=left  Value=TO
  Data Type Conversion1 : DataTypeConversion  DataType=boolean  SaturateOnIntegerOverflow=on
  Data Type Conversion2 : DataTypeConversion  DataType=double  SaturateOnIntegerOverflow=on
  Data Type Conversion3 : DataTypeConversion  DataType=boolean  SaturateOnIntegerOverflow=on
  Data Type Conversion5 : DataTypeConversion  DataType=double  SaturateOnIntegerOverflow=on
  Integrator : Integrator  ExternalReset=level
  Relational Operator : RelationalOperator  InputSameDT=on
  S-R Flip-Flop : simulink_extras/Flip Flops/S-R Flip-Flop  initial_condition=0
  Switch1 : Switch  Threshold=1  SaturateOnIntegerOverflow=on  InputSameDT=on
  Switch2 : Switch  Threshold=1  SaturateOnIntegerOverflow=on  InputSameDT=on
  Time elapse : Outport
  wires:
  Data Type Conversion5/1 -> Switch1/3
  S-R Flip-Flop/1 -> Data Type Conversion5/1
  Data Type Conversion2/1 -> Integrator/2
  S-R Flip-Flop/2 -> Data Type Conversion2/1
  Start/1 -> Data Type Conversion1/1
  Data Type Conversion1/1 -> S-R Flip-Flop/1
  Reset/1 -> Data Type Conversion3/1
  Data Type Conversion3/1 -> S-R Flip-Flop/2
  Switch2/1 -> Integrator/1
  Constant3/1 -> Relational Operator/2
  Constant1/1 -> Switch1/1, Switch2/3
  Integrator/1 -> Relational Operator/1
  Relational Operator/1 -> Switch1/2, Time elapse/1
  Switch1/1 -> Switch2/2
  Constant2/1 -> Switch2/1

== system qvmbocsh41_od_2/ABS Block/Signal Processing/ Wheel Accel./Deceleration ==
  r_eff : Inport
  Omega : Inport  Port=2
  Derivative : Derivative
  Low-pass filter : TransferFcn  Numerator=[1.15]  Denominator=[0.0105 1]
  Product2 : Product  Inputs=**  SaturateOnIntegerOverflow=on  InputSameDT=on
  To Workspace1 : ToWorkspace  VariableName=om_dot_per  SaveFormat=Array
      settings: MaxDataPoints=10000
  To Workspace3 : ToWorkspace  VariableName=om_dotcont  SaveFormat=Array
      settings: MaxDataPoints=10000
  Om_dot_periph. : Outport
  Om_dot_angul. : Outport  Port=2
  wires:
  Low-pass filter/1 -> Product2/2, Om_dot_angul./1  "om_dot"
  Derivative/1 -> Low-pass filter/1, To Workspace3/1  "dot"
  r_eff/1 -> Product2/1
  Omega/1 -> Derivative/1
  Product2/1 -> Om_dot_periph./1, To Workspace1/1

== system qvmbocsh41_od_2/ABS Block/Signal Processing/Om_dot / Om ==
  Om_dot : Inport
  Omega : Inport  Port=2
  Gain2 : Gain  Gain=-1  SaturateOnIntegerOverflow=on
  Product : Product  Inputs=*/  SaturateOnIntegerOverflow=on  InputSameDT=on
  Relational Operator1 : RelationalOperator  Operator=>  InputSameDT=on
  Threshold Value : Constant  Orientation=left  Value=om_dot_om
  To Workspace2 : ToWorkspace  VariableName=om_dotf_om  SaveFormat=Array
      settings: MaxDataPoints=10000
  Om_dot / Om : Outport
  wires:
  Threshold Value/1 -> Relational Operator1/2
  Product/1 -> Relational Operator1/1, To Workspace2/1
  Gain2/1 -> Product/1
  Om_dot/1 -> Gain2/1
  Relational Operator1/1 -> Om_dot / Om/1
  Omega/1 -> Product/2

== system qvmbocsh41_od_2/ABS Block/Signal Processing/Slip Threshold ==
  Om*r_eff : Inport
  X2_dot : Inport  Port=2
  " Slip Computation" : Fcn  Expr=1.0 - u(1)/u(2)
  Mux : Mux  Inputs=2
  Slip Comparator : RelationalOperator  Operator=>  InputSameDT=on
  Slip Comparator1 : RelationalOperator  Operator=>  InputSameDT=on
  Slip set-poit : Constant  Orientation=left  Value=0.01*Slip
  Slip set-poit1 : Constant  Orientation=left  Value=0.01*Slipmin
  To Workspace18 : ToWorkspace  VariableName=slip_est  SaveFormat=Array
      settings: MaxDataPoints=10000
  Comp. S-min : Outport
  Slip : Outport  Port=2
  Comp.Output : Outport  Port=3
  wires:
  Slip set-poit/1 -> Slip Comparator/2
  Mux/1 -> " Slip Computation"/1  "Vehicle-Wheel Vel."
  " Slip Computation"/1 -> To Workspace18/1, Slip Comparator/1, Slip/1, Slip Comparator1/1
  Om*r_eff/1 -> Mux/1
  Slip Comparator/1 -> Comp.Output/1  "Slip exceed"
  X2_dot/1 -> Mux/2
  Slip set-poit1/1 -> Slip Comparator1/2
  Slip Comparator1/1 -> Comp. S-min/1  "Slip exceed"

== system qvmbocsh41_od_2/ABS Block/Signal Processing/Subsystem1 ==
  In1 : Inport
  Logical Operator2 : Logic  Operator=XOR
  Logical Operator3 : Logic
  Memory : Memory
  Neg. Slope : Outport
  wires:
  Logical Operator3/1 -> Neg. Slope/1
  In1/1 -> Logical Operator2/2, Memory/1
  Logical Operator2/1 -> Logical Operator3/2
  Memory/1 -> Logical Operator3/1, Logical Operator2/1

== system qvmbocsh41_od_2/ABS Block/Signal Processing/Subsystem10 ==
  In1 : Inport
  Logical Operator2 : Logic  Operator=XOR
  Logical Operator3 : Logic
  Memory : Memory
  Neg. Slope : Outport
  wires:
  Logical Operator3/1 -> Neg. Slope/1
  In1/1 -> Logical Operator2/2, Memory/1
  Logical Operator2/1 -> Logical Operator3/2
  Memory/1 -> Logical Operator3/1, Logical Operator2/1

== system qvmbocsh41_od_2/ABS Block/Signal Processing/Subsystem11 ==
  In1 : Inport
  Logical Operator2 : Logic  Operator=XOR
  Logical Operator3 : Logic
  Memory : Memory
  Neg. Slope : Outport
  wires:
  Logical Operator3/1 -> Neg. Slope/1
  In1/1 -> Logical Operator2/2, Memory/1
  Logical Operator2/1 -> Logical Operator3/2
  Memory/1 -> Logical Operator3/1, Logical Operator2/1

== system qvmbocsh41_od_2/ABS Block/Signal Processing/Subsystem12 ==
  In1 : Inport
  Logical Operator2 : Logic  Operator=XOR
  Logical Operator3 : Logic
  Memory : Memory
  Pos. Slope : Outport
  wires:
  Logical Operator3/1 -> Pos. Slope/1
  In1/1 -> Logical Operator2/2, Memory/1, Logical Operator3/1
  Logical Operator2/1 -> Logical Operator3/2
  Memory/1 -> Logical Operator2/1

== system qvmbocsh41_od_2/ABS Block/Signal Processing/Subsystem13 ==
  In1 : Inport
  Logical Operator2 : Logic  Operator=XOR
  Logical Operator3 : Logic
  Memory : Memory
  Pos. Slope : Outport
  wires:
  Logical Operator3/1 -> Pos. Slope/1
  In1/1 -> Logical Operator2/2, Memory/1, Logical Operator3/1
  Logical Operator2/1 -> Logical Operator3/2
  Memory/1 -> Logical Operator2/1

== system qvmbocsh41_od_2/ABS Block/Signal Processing/Subsystem14 ==
  In1 : Inport
  Logical Operator2 : Logic  Operator=XOR
  Logical Operator3 : Logic
  Memory : Memory
  Neg. Slope : Outport
  wires:
  Logical Operator3/1 -> Neg. Slope/1
  In1/1 -> Logical Operator2/2, Memory/1
  Logical Operator2/1 -> Logical Operator3/2
  Memory/1 -> Logical Operator3/1, Logical Operator2/1

== system qvmbocsh41_od_2/ABS Block/Signal Processing/Subsystem3 ==
  In1 : Inport
  Logical Operator2 : Logic  Operator=XOR
  Logical Operator3 : Logic
  Memory : Memory
  Pos. Slope : Outport
  wires:
  Logical Operator3/1 -> Pos. Slope/1
  In1/1 -> Logical Operator2/2, Memory/1, Logical Operator3/1
  Logical Operator2/1 -> Logical Operator3/2
  Memory/1 -> Logical Operator2/1

== system qvmbocsh41_od_2/ABS Block/Signal Processing/Subsystem5 ==
  In1 : Inport
  Logical Operator2 : Logic  Operator=XOR
  Logical Operator3 : Logic
  Memory : Memory
  Pos. Slope : Outport
  wires:
  Logical Operator3/1 -> Pos. Slope/1
  In1/1 -> Logical Operator2/2, Memory/1, Logical Operator3/1
  Logical Operator2/1 -> Logical Operator3/2
  Memory/1 -> Logical Operator2/1

== system qvmbocsh41_od_2/ABS Block/Signal Processing/Subsystem7 ==
  In1 : Inport
  Logical Operator2 : Logic  Operator=XOR
  Logical Operator3 : Logic
  Memory : Memory
  Neg. Slope : Outport
  wires:
  Logical Operator3/1 -> Neg. Slope/1
  In1/1 -> Logical Operator2/2, Memory/1
  Logical Operator2/1 -> Logical Operator3/2
  Memory/1 -> Logical Operator3/1, Logical Operator2/1

== system qvmbocsh41_od_2/ABS Block/Signal Processing/Subsystem8 ==
  In1 : Inport
  Logical Operator2 : Logic  Operator=XOR
  Logical Operator3 : Logic
  Memory : Memory
  Neg. Slope : Outport
  wires:
  Logical Operator3/1 -> Neg. Slope/1
  In1/1 -> Logical Operator2/2, Memory/1
  Logical Operator2/1 -> Logical Operator3/2
  Memory/1 -> Logical Operator3/1, Logical Operator2/1

== system qvmbocsh41_od_2/ABS Block/Signal Processing/Subsystem9 ==
  In1 : Inport
  Logical Operator2 : Logic  Operator=XOR
  Logical Operator3 : Logic
  Memory : Memory
  Pos. Slope : Outport
  wires:
  Logical Operator3/1 -> Pos. Slope/1
  In1/1 -> Logical Operator2/2, Memory/1, Logical Operator3/1
  Logical Operator2/1 -> Logical Operator3/2
  Memory/1 -> Logical Operator2/1

== system qvmbocsh41_od_2/ABS Block/Signal Processing/Threshold  A, +a ==
  Om_dot_periph. : Inport
  +a Comparator1 : RelationalOperator  Operator=>  InputSameDT=on
  +a positive acc. : Constant  Orientation=left  Value=pos_a
  A Comparator : RelationalOperator  Operator=>  InputSameDT=on
  A positive acc. : Constant  Orientation=left  Value=A
  " > A" : Outport
  > +a : Outport  Port=2
  wires:
  +a Comparator1/1 -> > +a/1
  +a positive acc./1 -> +a Comparator1/2
  A Comparator/1 -> " > A"/1
  A positive acc./1 -> A Comparator/2
  Om_dot_periph./1 -> A Comparator/1, +a Comparator1/1

== system qvmbocsh41_od_2/ABS Block/Signal Processing/Threshold -a ==
  Om_dot_periph. : Inport
  -a Comparator1 : RelationalOperator  InputSameDT=on
  -a negative acc. : Constant  Orientation=left  Value=neg_a
  Gain2 : Gain  Gain=-1  SaturateOnIntegerOverflow=on
  > -a : Outport
  wires:
  Gain2/1 -> -a Comparator1/1
  -a Comparator1/1 -> > -a/1
  -a negative acc./1 -> -a Comparator1/2
  Om_dot_periph./1 -> Gain2/1

== system qvmbocsh41_od_2/ABS Block/Subsystem/Generator ==
  In : Inport
  Constant1 : Constant  Orientation=left  Value=0
  Data Type Conversion1 : DataTypeConversion  DataType=boolean  SaturateOnIntegerOverflow=on
  Data Type Conversion2 : DataTypeConversion  Orientation=left  DataType=double  SaturateOnIntegerOverflow=on
  Data Type Conversion5 : DataTypeConversion  DataType=boolean  SaturateOnIntegerOverflow=on
  Logical Operator2 : Logic  Operator=OR
  Memory1 : Memory  Orientation=left
  Memory2 : Memory  Orientation=left
  Subsystem2 : Subsystem
  Switch2 : Switch  Threshold=1  SaturateOnIntegerOverflow=on  InputSameDT=on
  Timer R1 : Subsystem  mask{TC=TC}
      mask prompts: TC "Cycle Time [s]"
  Timer R2 : Subsystem  mask{TO=TO}
      mask prompts: TO "Open time [s]"
  Out : Outport
  wires:
  Timer R2/1(Time elapse) -> Out/1
  Data Type Conversion2/1 -> Switch2/1
  Data Type Conversion1/1 -> Logical Operator2/2
  Constant1/1 -> Switch2/3
  Memory2/1 -> Data Type Conversion2/1
  Switch2/1 -> Data Type Conversion1/1
  Memory1/1 -> Memory2/1, Timer R2/2(Reset), Timer R1/2(Reset)
  Data Type Conversion5/1 -> Switch2/2, Subsystem2/1(In1)
  Subsystem2/1(Pos. Slpoe) -> Logical Operator2/1
  In/1 -> Data Type Conversion5/1
  Timer R1/1(Time elapse) -> Memory1/1
  Logical Operator2/1 -> Timer R1/1(Start), Timer R2/1(Start)

== system qvmbocsh41_od_2/ABS Block/Subsystem/One Cycle Indicator ==
  In : Inport
  Logical Operator3 : Logic  Operator=OR
  Memory : Memory
  S-R Flip-Flop : simulink_extras/Flip Flops/S-R Flip-Flop  Orientation=left  initial_condition=0
  Terminator : Terminator
  Q : Outport
  wires:
  S-R Flip-Flop/2 -> Terminator/1
  In/1 -> Logical Operator3/2
  S-R Flip-Flop/1 -> Memory/1
  Memory/1 -> Q/1, Logical Operator3/1
  Logical Operator3/1 -> S-R Flip-Flop/1

== system qvmbocsh41_od_2/ABS Block/Subsystem/Generator/Subsystem2 ==
  In1 : Inport
  Logical Operator2 : Logic  Operator=XOR
  Logical Operator3 : Logic
  Memory : Memory
  Pos. Slpoe : Outport
  wires:
  Logical Operator3/1 -> Pos. Slpoe/1
  In1/1 -> Logical Operator3/1, Memory/1, Logical Operator2/2
  Logical Operator2/1 -> Logical Operator3/2
  Memory/1 -> Logical Operator2/1

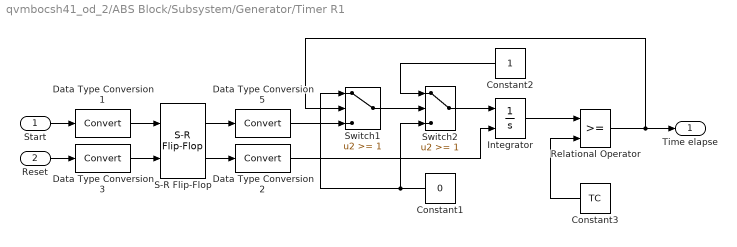
== system qvmbocsh41_od_2/ABS Block/Subsystem/Generator/Timer R1 ==
  Start : Inport
  Reset : Inport  Port=2
  Constant1 : Constant  Orientation=left  Value=0
  Constant2 : Constant  Orientation=left
  Constant3 : Constant  Orientation=left  Value=TC
  Data Type Conversion1 : DataTypeConversion  DataType=boolean  SaturateOnIntegerOverflow=on
  Data Type Conversion2 : DataTypeConversion  DataType=double  SaturateOnIntegerOverflow=on
  Data Type Conversion3 : DataTypeConversion  DataType=boolean  SaturateOnIntegerOverflow=on
  Data Type Conversion5 : DataTypeConversion  DataType=double  SaturateOnIntegerOverflow=on
  Integrator : Integrator  ExternalReset=level
  Relational Operator : RelationalOperator  InputSameDT=on
  S-R Flip-Flop : simulink_extras/Flip Flops/S-R Flip-Flop  initial_condition=0
  Switch1 : Switch  Threshold=1  SaturateOnIntegerOverflow=on  InputSameDT=on
  Switch2 : Switch  Threshold=1  SaturateOnIntegerOverflow=on  InputSameDT=on
  Time elapse : Outport
  wires:
  Data Type Conversion5/1 -> Switch1/3
  S-R Flip-Flop/1 -> Data Type Conversion5/1
  Data Type Conversion2/1 -> Integrator/2
  S-R Flip-Flop/2 -> Data Type Conversion2/1
  Start/1 -> Data Type Conversion1/1
  Data Type Conversion1/1 -> S-R Flip-Flop/1
  Reset/1 -> Data Type Conversion3/1
  Data Type Conversion3/1 -> S-R Flip-Flop/2
  Switch2/1 -> Integrator/1
  Constant3/1 -> Relational Operator/2
  Constant1/1 -> Switch1/1, Switch2/3
  Integrator/1 -> Relational Operator/1
  Relational Operator/1 -> Switch1/2, Time elapse/1
  Switch1/1 -> Switch2/2
  Constant2/1 -> Switch2/1

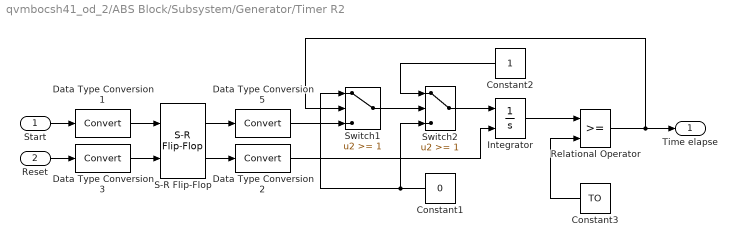
== system qvmbocsh41_od_2/ABS Block/Subsystem/Generator/Timer R2 ==
  Start : Inport
  Reset : Inport  Port=2
  Constant1 : Constant  Orientation=left  Value=0
  Constant2 : Constant  Orientation=left
  Constant3 : Constant  Orientation=left  Value=TO
  Data Type Conversion1 : DataTypeConversion  DataType=boolean  SaturateOnIntegerOverflow=on
  Data Type Conversion2 : DataTypeConversion  DataType=double  SaturateOnIntegerOverflow=on
  Data Type Conversion3 : DataTypeConversion  DataType=boolean  SaturateOnIntegerOverflow=on
  Data Type Conversion5 : DataTypeConversion  DataType=double  SaturateOnIntegerOverflow=on
  Integrator : Integrator  ExternalReset=level
  Relational Operator : RelationalOperator  InputSameDT=on
  S-R Flip-Flop : simulink_extras/Flip Flops/S-R Flip-Flop  initial_condition=0
  Switch1 : Switch  Threshold=1  SaturateOnIntegerOverflow=on  InputSameDT=on
  Switch2 : Switch  Threshold=1  SaturateOnIntegerOverflow=on  InputSameDT=on
  Time elapse : Outport
  wires:
  Data Type Conversion5/1 -> Switch1/3
  S-R Flip-Flop/1 -> Data Type Conversion5/1
  Data Type Conversion2/1 -> Integrator/2
  S-R Flip-Flop/2 -> Data Type Conversion2/1
  Start/1 -> Data Type Conversion1/1
  Data Type Conversion1/1 -> S-R Flip-Flop/1
  Reset/1 -> Data Type Conversion3/1
  Data Type Conversion3/1 -> S-R Flip-Flop/2
  Switch2/1 -> Integrator/1
  Constant3/1 -> Relational Operator/2
  Constant1/1 -> Switch1/1, Switch2/3
  Integrator/1 -> Relational Operator/1
  Relational Operator/1 -> Switch1/2, Time elapse/1
  Switch1/1 -> Switch2/2
  Constant2/1 -> Switch2/1
